simulink model "w1"  (R2020b)
settings: Solver=VariableStepAuto  StartTime=0.0  StopTime=10  MaxStep=0.0001  RelTol=1e-3
InitFcn:
  | m=0.5;
  | c=sqrt(2);
  | k=1;
  | w=sqrt(k/m);
  | kes=c/(2*w*m);
settings Model: Creator=雨后星空  LastModifiedBy=雨后星空

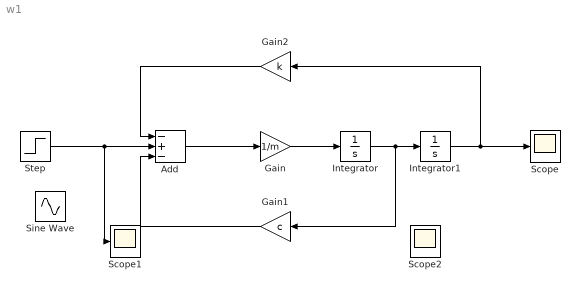
== system w1 ==
  Add : Sum  Inputs=-+-
  Gain : Gain  Gain=1/m
  Gain1 : Gain  Gain=c
  Gain2 : Gain  Gain=k
  Integrator : Integrator
  Integrator1 : Integrator
  Scope : Scope
  Scope1 : Scope
  Scope2 : Scope
  Sine Wave : Sin  SampleTime=0
  Step : Step  SampleTime=0
  wires:
  Add/1 -> Gain/1
  Gain/1 -> Integrator/1
  Integrator/1 -> Gain1/1, Integrator1/1
  Integrator1/1 -> Gain2/1, Scope/1
  Gain2/1 -> Add/1
  Gain1/1 -> Add/3
  Step/1 -> Scope1/1, Add/2
